simulink model "step11"  (R2016b)
settings: Solver=VariableStepAuto  StartTime=0.0  StopTime=30  RelTol=1e-3
values from neighbouring files (symbols this model uses):
  A = [0 1 0 0 ... (first row only)    [EE547FinalProject.m]
  B = [0;B1;0;B2]    [EE547FinalProject.m]
  C = [1 0 0 0; 0 1 0 0; 0 0 1 0; 0 0 0 1]    [EE547FinalProject.m]
  D = zeros(size(C,1),size(B,2))    [EE547FinalProject.m]
  gainL = place(transpose(A), transpose(C), pole_obser)'    [EE547FinalProject.m]
  xhatini = [0 0 0 0]    [EE547FinalProject.m]
  xini = [0 0 0 0]    [EE547FinalProject.m]
settings Model: Creator=muller  LastModifiedBy=muller

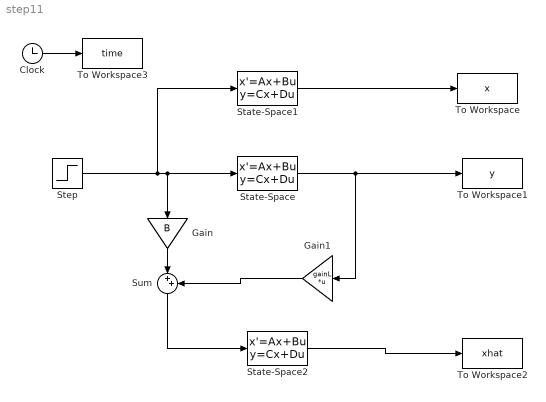
== system step11 ==
  Clock : Clock
  Gain : Gain  Gain=B
  Gain1 : Gain  Gain=gainL  Multiplication=Matrix(K*u)
  State-Space : StateSpace  A=A  B=B  C=C  D=D  X0=xini
  State-Space1 : StateSpace  A=A  B=B  C=eye(4)  D=zeros(size(C,1),1)  X0=xini
  State-Space2 : StateSpace  A=A-gainL*C  B=eye(4)  C=eye(4)  D=zeros(4)  X0=xhatini
  Step : Step  SampleTime=0
  Sum : Sum  Inputs=|++
  To Workspace : ToWorkspace  VariableName=x  SampleTime=-1
  To Workspace1 : ToWorkspace  VariableName=y  SampleTime=-1
  To Workspace2 : ToWorkspace  VariableName=xhat  SampleTime=-1
  To Workspace3 : ToWorkspace  VariableName=time  SampleTime=-1
  wires:
  Clock/1 -> To Workspace3/1
  State-Space1/1 -> To Workspace/1
  State-Space/1 -> Gain1/1, To Workspace1/1
  State-Space2/1 -> To Workspace2/1
  Step/1 -> Gain/1, State-Space/1, State-Space1/1
  Gain/1 -> Sum/1
  Sum/1 -> State-Space2/1
  Gain1/1 -> Sum/2
